simulink model "donghocnguoc_vantoc_2019"  (R2023b)
settings: Solver=FixedStepAuto  StartTime=0.0  StopTime=6  FixedStep=0.01  RelTol=1e-3
settings Model: Creator=DELL  LastModifiedBy=DELL

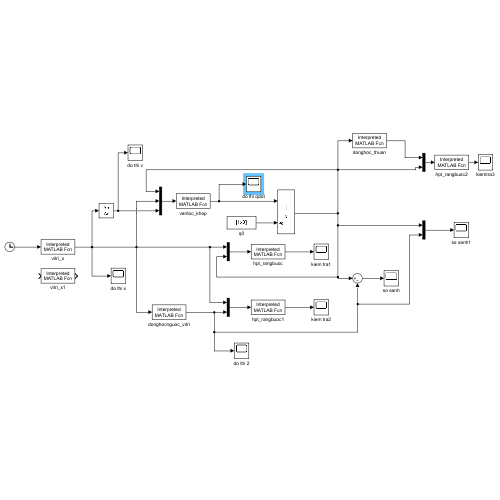
[thumbnail: Simulink's stored preview of the top-level diagram]
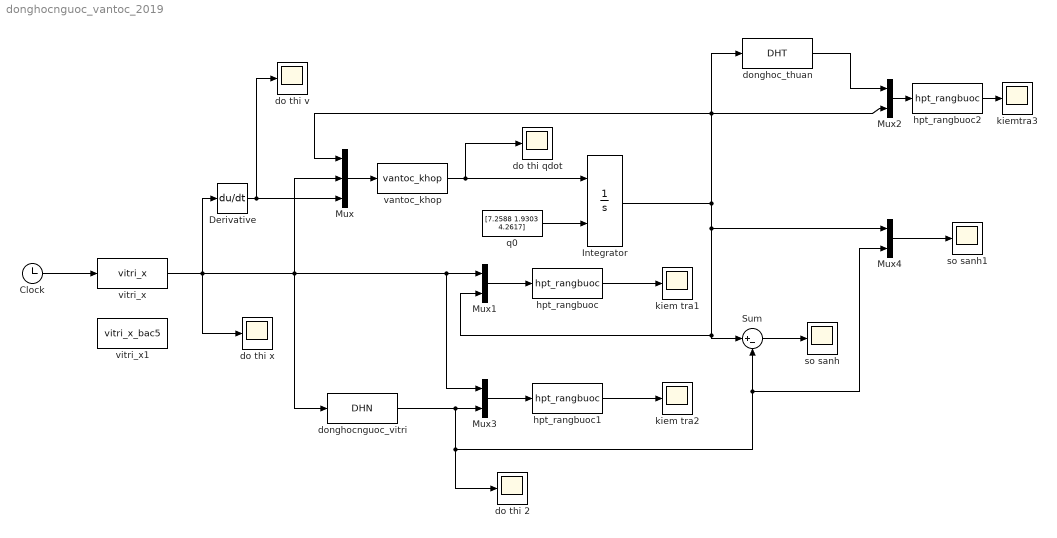
== system donghocnguoc_vantoc_2019 ==
  Clock : Clock
      settings: Decimation=2
  Derivative : Derivative
  Integrator : Integrator  InitialConditionSource=external
  Mux : Mux  Inputs=3
  Mux{1..4} (4 alike) : Mux  Inputs=2
  Sum : Sum  Inputs=|+-
  do thi 2 : Scope
  do thi qdot : Scope
  do thi v : Scope
  do thi x : Scope
  donghoc_thuan : MATLABFcn  MATLABFcn=DHT  OutputDimensions=3  OutputSignalType=real  Output1D=off
  donghocnguoc_vitri : MATLABFcn  MATLABFcn=DHN  OutputDimensions=3  OutputSignalType=real  Output1D=off
  hpt_rangbuoc : MATLABFcn  MATLABFcn=hpt_rangbuoc
  hpt_rangbuoc1 : MATLABFcn  MATLABFcn=hpt_rangbuoc
  hpt_rangbuoc2 : MATLABFcn  MATLABFcn=hpt_rangbuoc
  kiem tra1 : Scope
  kiem tra2 : Scope
  kiemtra3 : Scope
  q0 : Constant  Value="[7.2588    1.9303    4.2617]"
  so sanh : Scope
  so sanh1 : Scope
  vantoc_khop : MATLABFcn  MATLABFcn=vantoc_khop  OutputDimensions=3  OutputSignalType=real  Output1D=off
  vitri_x : MATLABFcn  MATLABFcn=vitri_x  OutputDimensions=3
  vitri_x1 : MATLABFcn  MATLABFcn=vitri_x_bac5  OutputDimensions=3
  wires:
  vantoc_khop/1 -> do thi qdot/1, Integrator/1
  Integrator/1 -> Mux1/2, Sum/1, Mux4/1, donghoc_thuan/1, Mux2/2, Mux/1
  Mux/1 -> vantoc_khop/1
  Clock/1 -> vitri_x/1
  hpt_rangbuoc/1 -> kiem tra1/1
  q0/1 -> Integrator/2
  vitri_x/1 -> Mux/2, donghocnguoc_vitri/1, Mux1/1, Mux3/1, do thi x/1, Derivative/1
  Mux1/1 -> hpt_rangbuoc/1
  hpt_rangbuoc1/1 -> kiem tra2/1
  Mux3/1 -> hpt_rangbuoc1/1
  donghocnguoc_vitri/1 -> Sum/2, Mux4/2, do thi 2/1, Mux3/2
  Derivative/1 -> Mux/3, do thi v/1
  Sum/1 -> so sanh/1
  donghoc_thuan/1 -> Mux2/1
  hpt_rangbuoc2/1 -> kiemtra3/1
  Mux2/1 -> hpt_rangbuoc2/1
  Mux4/1 -> so sanh1/1
